simulink model "Steering_dynamics_discrete_mdl"  (R2026a)
settings: Solver=VariableStepAuto  StopTime=1
undefined symbols (not defined in the file): Vehicle
(part 1 of 2)
settings Model: PacingRate=0.500000  Creator=irfan  LastModifiedBy=irfan

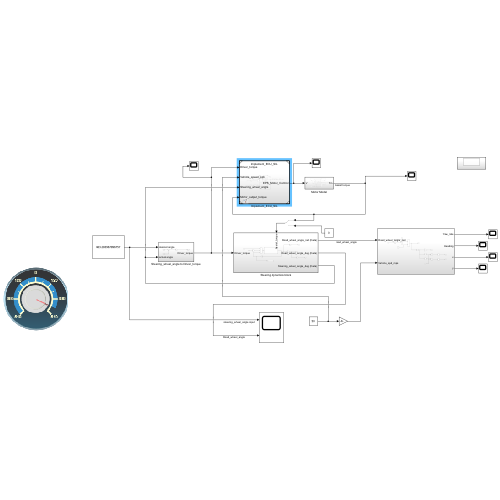
[thumbnail: Simulink's stored preview of the top-level diagram]
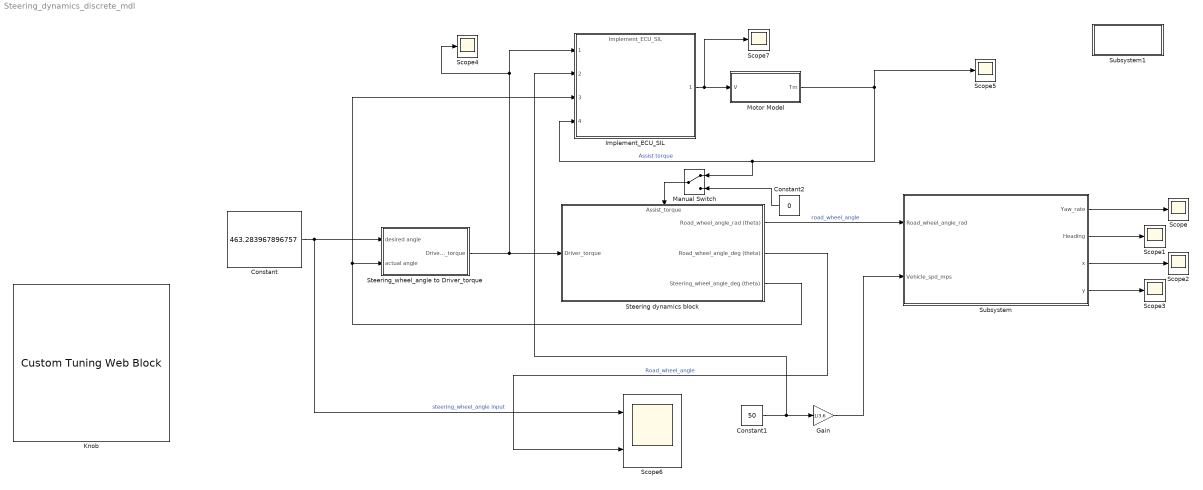
== system Steering_dynamics_discrete_mdl ==
  Constant : Constant  Value=463.283967896757
  Constant1 : Constant  Value=50
  Constant2 : Constant  Value=0
  Gain : Gain  Gain=1/3.6
  Implement_ECU_SIL : ModelReference  ModelNameDialog=Implement_ECU_SIL.slx  SimulationMode=Normal  ModelReferenceVersion=1.136
  Knob : CustomTuningWebBlock  LabelPosition=Hide  ShowInitialText=on  Configuration="{\"components\":[{\"name\":\"CircularScaleComponent\",\"settings\":{\"bounds\":{\"max\":540,\"min\":-540,\"tickInterval\":90},\"direction\":\"cw\",\"flipLimits\":0,\"innerRadius\":0.6636618227670849,\"internalTickHeightScaleFactor\":1,\"labelColor\":[255,255,200],\"labelFont\":{\"font\":\"Arial\",\"fontSize\":12},\"labelRadius\":0.79,\"labelTransparency\":1,\"minorTickHeightScaleFactor\":0.2,\"needleImage\":{\"size\":[150,150],\"src\":\"data:image\\/svg+xml;base64,PD94bWwgdmVyc2lvbj0iMS4wIiBlbmNvZGluZz0idXRmLTgiPz4NCjwhLS0gR2VuZXJhdG9yOiBBZG9iZSBJbGx1c3RyYXRvciAyNS4yLjMsIFNWRyBFeHBvcnQgUGx1Zy1JbiAuIFNWRyBWZXJzaW9uOiA2LjAwIEJ1aWxkIDApICAtLT4NCjxzdmcgdmVyc2lvbj0iMS4xIiBpZD0iTGF5ZXJfMSIgeG1sbnM9Imh0dHA6Ly93d3cudzMub3JnLzIwMDAvc3ZnIiB4bWxuczp4bGluaz0iaHR0cDovL3d3dy53My5vcmcvMTk5OS94bGluayIgeD0iMHB4IiB5PSIwcHgiDQoJIHZpZXdCb3g9IjAgMCAxNTIgMTUyIiBzdHlsZT0iZW5hYmxl ...(+37472 chars)\"},\"needleOffset\":[0,0],\"needleOrientation\":-45,\"needleRotation\":90,\"needleSize\":{\"height\":0.44,\"width\":0.44},\"outerRadius\":0.5053386200069245,\"position\":[0,0,1,1],\"referencePoint\":\"auto\",\"scaleAngle\":270,\"scaleAngleOffset\":135,\"scaleColors\":[],\"scaleColorsSize\":0.2,\"scaleDirection\":\"CW\",\"scalePosition\":[0,0,1,1],\"showLabels\":1,\"showMinorTicks\":1,\"showSpanLine\":true,\"showTicks\":1,\"tickColor\":[252,252,197],\"tickTransparency\":1,\"valueBarColor\":[0,114,189],\"valueBarPosition\":[0,0,1,1],\"valueBarSize\":0.2,\"valueBarTransparency\":1}},{\"name\":\"BackgroundImageComponent\",\"settings\":{\"image\":{\"size\":[385,373],\"src\":\"data:image\\/svg+xml;base64,PD94bWwgdmVyc2lvbj0iMS4wIiBlbmNvZGluZz0idXRmLTgiPz4NCjwhLS0gR2VuZXJhdG9yOiBBZG9iZSBJbGx1c3RyYXRvciAyNS4wLjAsIFNWRyBFeHBvcnQgUGx1Zy1JbiAuIFNWRyBWZXJzaW9uOiA2LjAwIEJ1aWxkIDApICAtLT4NCjxzdmcgdmVyc2lvbj0iMS4xIg0KCSBpZD0iTGF5ZXJfMl8xXyIgeG1sbnM6Y2M9Imh0dHA6Ly9jcmVhdGl2ZWNvbW1vbnMub3JnL25zIyIgeG1sbnM6ZGM9Imh0dHA6Ly9wdXJsLm9yZy9kYy9lbGVtZW50cy8xLjEvIiB4bWxuczppbmtzY2FwZT0iaHR0cDovL3d3dy5pbmtzY2FwZS5vcmcv ...(+4184 chars)\",\"srcOrientation\":\"horizontal\"},\"position\":[0,0,1,1],\"scaleMode\":\"0\"}},{\"name\":\"ForegroundImageComponent\",\"settings\":{\"image\":{\"size\":[0,0],\"src\":\"default\",\"srcOrientation\":[]},\"isForeground\":1,\"position\":[0,0,1,1],\"scaleMode\":\"0\"}}],\"derived\":{\"blockParameters\":{\"ForegroundColor\":[0.9882352941176471,0.9882352941176471,0.7725490196078432],\"Limits\":{\"Max\":540,\"Min\":-540,\"Ticks\":90},\"ScaleColors\":[],\"ScaleDirection\":\"Clockwise\",\"ScaleMax\":540,\"ScaleMin\":-540,\"TickInterval\":90,\"fixedAspectRatio\":\"on\"}},\"settings\":{\"BindingType\":\"param\",\"aspectRatio\":1,\"backgroundColor\":[0,0,0,\"1\"],\"backgroundOffset\":1,\"backgroundOpacity\":1,\"direction\":\"cw\",\"fixedAspectRatio\":\"on\",\"flipLimits\":0,\"foregroundColor\":[252,252,196],\"orientation\":\"horizontal\",\"showBackgroundColor\":false,\"value\":0,\"version\":\"R2023a\"},\"type\":\"CircularGauge\"}"
  Manual Switch : ManualSwitch
  Motor Model : Subsystem
  Scope{,1..5,7} (7 alike) : Scope
      Scope settings: ActiveDisplayYMinimum=-0.41852969068965112  ActiveDisplayYMaximum=0.41898071432653589
      Scope1 settings: ActiveDisplayYMinimum=-2960.1657546851284  ActiveDisplayYMaximum=1945.8517097629976
      Scope2 settings: ActiveDisplayYMinimum=-11.797897167685495  ActiveDisplayYMaximum=93.1218501417316  DataLoggingVariableName=ScopeData2
      Scope3 settings: ActiveDisplayYMinimum=-24.67380318583777  ActiveDisplayYMaximum=222.05922897318413  DataLoggingVariableName=ScopeData3
      Scope4 settings: ActiveDisplayYMinimum=-49.713057986087165  ActiveDisplayYMaximum=66.391641557951161  DataLoggingVariableName=ScopeData4
      Scope5 settings: ActiveDisplayYMinimum=-0.50378714090280319  ActiveDisplayYMaximum=2.7744336390259794  DataLoggingVariableName=ScopeData5
      Scope7 settings: ActiveDisplayYMinimum=-1.4999999999999996  ActiveDisplayYMaximum=13.5  DataLoggingVariableName=ScopeData7
  Scope6 : Scope  NumInputPorts=2
      settings: ActiveDisplayYMinimum=-293.12107836101222  ActiveDisplayYMaximum=566.53072227155849  DataLoggingVariableName=ScopeData6
  Steering dynamics block : Subsystem
      settings: PortSchema="{\"entries\":[{\"content\":{\"sides\":[{\"content\":{\"connectorIds\":[\"In1\"]},\"type\":\"ConnectorPlacement.EquallySpacedRectSide\",\"uuid\":\"f34f9e01-3985-4939-b31b-584f55462760\"},{\"content\":{\"connectorIds\":[\"Out1\",\"Out2\",\"Out3\"],\"side\":\"RIGHT\"},\"type\":\"ConnectorPlacement.EquallySpacedRectSide\",\"uuid\":\"65e82b14-232b-4b0e-9346-951018240c67\"},{\"content\":{\"connectorIds\":[\"In2\"],\"side\":\"TOP\"},\"type\":\"ConnectorPlacement.EquallySpacedRectSide\",\"uuid\":\"bb91e0e5-5fa0-49d2-9d07-33e334c3a6bc\"}]},\"type\":\"ConnectorPlacement.EquallySpacedConnector\",\"uuid\":\"c6d9befd-20cf-40bb-aaee-7c6c46e18759\"}],\"packageUris\":[\"http://schema.mathworks.com/mf0/Connector/R2020b\"],\"version\":\"1.0\"}"
  Steering_wheel_angle to Driver_torque : Subsystem
  Subsystem : Subsystem
  Subsystem1 : Subsystem
  wires:
  Constant/1 -> Scope6/1, Steering_wheel_angle to Driver_torque/1(desired angle)  "steering_wheel_angle input"
  Steering_wheel_angle to Driver_torque/1(Driver_torque) -> Steering dynamics block/1(Driver_torque), Implement_ECU_SIL/1, Scope4/1
  Steering dynamics block/3(Steering_wheel_angle_deg (theta)) -> Implement_ECU_SIL/3, Steering_wheel_angle to Driver_torque/2(actual angle)
  Steering dynamics block/1(Road_wheel_angle_rad (theta)) -> Subsystem/1(Road_wheel_angle_rad)  "road_wheel_angle"
  Constant1/1 -> Implement_ECU_SIL/2, Gain/1
  Gain/1 -> Subsystem/2(Vehicle_spd_mps)
  Subsystem/1(Yaw_rate) -> Scope/1
  Subsystem/2(Heading) -> Scope1/1
  Subsystem/3(x) -> Scope2/1
  Subsystem/4(y) -> Scope3/1
  Steering dynamics block/2(Road_wheel_angle_deg (theta)) -> Scope6/2  "Road_wheel_angle"
  Motor Model/1(Tm) -> Implement_ECU_SIL/4, Manual Switch/1, Scope5/1  "Assist torque"
  Implement_ECU_SIL/1 -> Scope7/1, Motor Model/1(V)
  Manual Switch/1 -> Steering dynamics block/2(Assist_torque)
  Constant2/1 -> Manual Switch/2

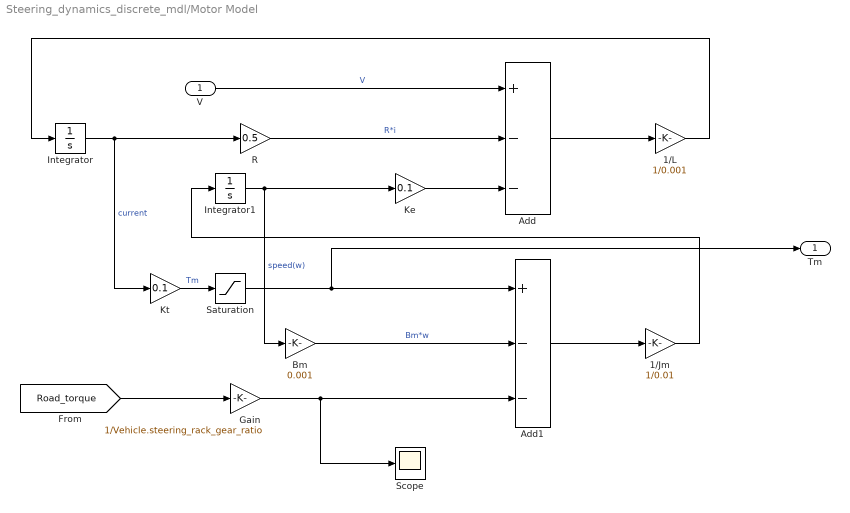
== system Steering_dynamics_discrete_mdl/Motor Model ==
  V : Inport
  1/Jm : Gain  Gain=1/0.01
  1/L : Gain  Gain=1/0.001
  Add : Sum  Inputs=+--
  Add1 : Sum  Inputs=+--
  Bm : Gain  Gain=0.001
  Gain : Gain  Gain=1/Vehicle.steering_rack_gear_ratio
  Integrator : Integrator
  Integrator1 : Integrator
  Ke : Gain  Gain=0.1
  Kt : Gain  Gain=0.1
  R : Gain  Gain=0.5
  Saturation : Saturate  UpperLimit=40  LowerLimit=-40
  Scope : Scope
      settings: ActiveDisplayYMinimum=-0.14247771255001759  ActiveDisplayYMaximum=1.2822994129501586  DataLoggingVariableName=ScopeData13
  Tm : Outport
  wires:
  V/1 -> Add/1  "V"
  Integrator/1 -> Kt/1, R/1  "current"
  R/1 -> Add/2  "R*i"
  Integrator1/1 -> Ke/1, Bm/1  "speed(w)"
  Ke/1 -> Add/3
  Add/1 -> 1/L/1
  1/L/1 -> Integrator/1
  Kt/1 -> Saturation/1  "Tm"
  Bm/1 -> Add1/2  "Bm*w"
  Add1/1 -> 1/Jm/1
  1/Jm/1 -> Integrator1/1
  [Road_torque] -> Gain/1
  Gain/1 -> Scope/1, Add1/3
  Saturation/1 -> Tm/1, Add1/1
